simulink model "simulador_Ref"  (R2020b)
settings: Solver=ode1  StartTime=0.0  StopTime=T_end  FixedStep=0.01  RelTol=1e-3
values from neighbouring files (symbols this model uses):
  a = 1.4/255    (= 0.00549019607843)    [main_01.m]
  b = 0.03    [main_01.m]
  Ki = 10    [main_01.m]
  Kp = 30    [main_01.m]
  Ref = 36    [main_01.m]
  T_amb = 29.63    [main_01.m]
  T_ini = 27.59    [main_01.m]
settings Model: Creator=nobel  LastModifiedBy=rober

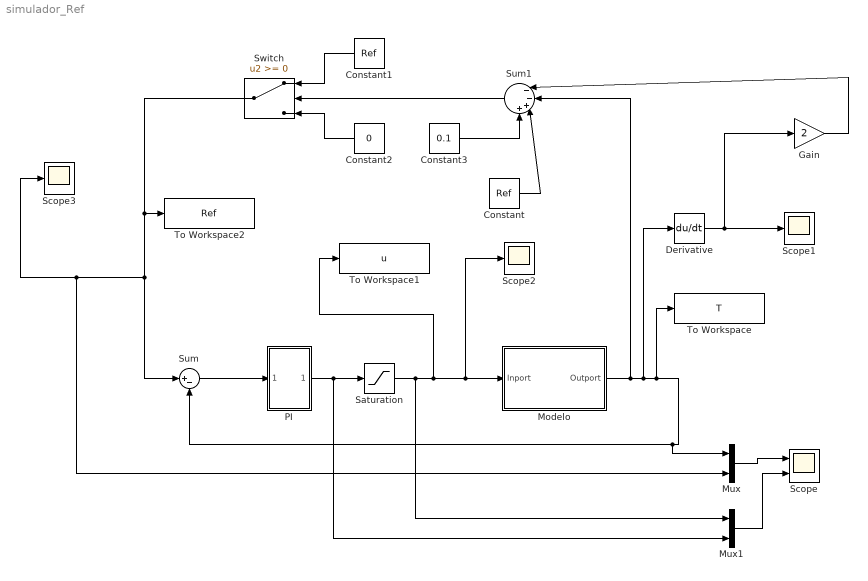
== system simulador_Ref ==
  Constant : Constant  Value=Ref
  Constant1 : Constant  Value=Ref
  Constant2 : Constant  Value=0
  Constant3 : Constant  Value=0.1
  Derivative : Derivative
  Gain : Gain  Gain=2
  Modelo : Subsystem
  Mux : Mux  Inputs=2
  Mux1 : Mux  Inputs=2
  PI : Subsystem
  Saturation : Saturate  UpperLimit=255  LowerLimit=0
  Scope : Scope  NumInputPorts=2
  Scope1 : Scope
  Scope2 : Scope
  Scope3 : Scope
  Sum : Sum  Inputs=|+-
  Sum1 : Sum  Inputs=|--++
  Switch : Switch
  To Workspace : ToWorkspace  VariableName=T  SampleTime=-1
  To Workspace1 : ToWorkspace  VariableName=u  SampleTime=-1
  To Workspace2 : ToWorkspace  VariableName=Ref  SampleTime=-1
  wires:
  Modelo/1(Outport) -> Sum1/2, Derivative/1, To Workspace/1, Mux/1, Sum/2
  Saturation/1 -> Mux1/1, To Workspace1/1, Scope2/1, Modelo/1(Inport)
  Sum/1 -> PI/1(In1)
  PI/1(Out1) -> Mux1/2, Saturation/1
  Derivative/1 -> Gain/1, Scope1/1
  Constant/1 -> Sum1/3
  Sum1/1 -> Switch/2
  Constant1/1 -> Switch/1
  Constant2/1 -> Switch/3
  Switch/1 -> To Workspace2/1, Mux/2, Scope3/1, Sum/1
  Constant3/1 -> Sum1/4
  Mux/1 -> Scope/1
  Gain/1 -> Sum1/1
  Mux1/1 -> Scope/2

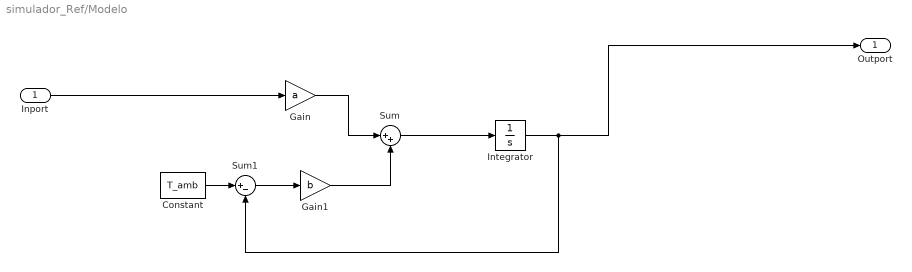
== system simulador_Ref/Modelo ==
  Inport : Inport
  Constant : Constant  Value=T_amb
  Gain : Gain  Gain=a
  Gain1 : Gain  Gain=b
  Integrator : Integrator  InitialCondition=T_ini
  Sum : Sum  Inputs=|++
  Sum1 : Sum  Inputs=|+-
  Outport : Outport
  wires:
  Inport/1 -> Gain/1
  Constant/1 -> Sum1/1
  Gain/1 -> Sum/1
  Gain1/1 -> Sum/2
  Sum1/1 -> Gain1/1
  Sum/1 -> Integrator/1
  Integrator/1 -> Outport/1, Sum1/2

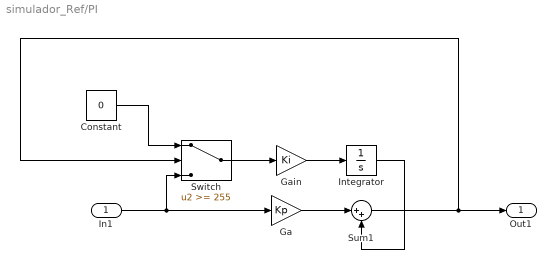
== system simulador_Ref/PI ==
  In1 : Inport
  Constant : Constant  Value=0
  Ga : Gain  Gain=Kp
  Gain : Gain  Gain=Ki
  Integrator : Integrator
  Sum1 : Sum  Inputs=|++
  Switch : Switch  Threshold=255
  Out1 : Outport
  wires:
  Ga/1 -> Sum1/1
  Sum1/1 -> Switch/2, Out1/1
  Gain/1 -> Integrator/1
  In1/1 -> Switch/3, Ga/1
  Integrator/1 -> Sum1/2
  Switch/1 -> Gain/1
  Constant/1 -> Switch/1
